simulink model "Matrix1_PP"  (Simulink 9.0)
settings: Solver=FixedStepDiscrete  StartTime=0.0  StopTime=19800  FixedStep=200  RelTol=1e-3  EnableMultiTasking=on
model workspace (MAT data in the model file):
  already_pp = 1
  input_dataset = Simulink.SimulationData.Dataset
  input_dataset.any.Name = ''
  input_dataset.any.Version = 3
  input_dataset.any.Storage = Simulink.SimulationData.Storage.RamDatasetStorage
  input_dataset.any.Storage.any.Version = 2
  input_dataset.any.Storage.any.Elements{1} = Simulink.SimulationData.Signal
  input_dataset.any.Storage.any.Elements{1}.Version = 1
  input_dataset.any.Storage.any.Elements{1}.Values = timeseries
  input_dataset.any.Storage.any.Elements{1}.Values.Name = 'unnamed'
  input_dataset.any.Storage.any.Elements{1}.Values.DataInfo = tsdata.datametadata
  input_dataset.any.Storage.any.Elements{1}.Values.DataInfo.Interpolation = tsdata.interpolation
  input_dataset.any.Storage.any.Elements{1}.Values.DataInfo.Interpolation.Fhandle : function handle (value not decoded)
  input_dataset.any.Storage.any.Elements{1}.Values.DataInfo.Interpolation.Name = 'linear'
  input_dataset.any.Storage.any.Elements{1}.Values.TimeInfo = tsdata.timemetadata
  input_dataset.any.Storage.any.Elements{1}.Values.TimeInfo.Length = 100
  input_dataset.any.Storage.any.Elements{1}.Values.TimeInfo.DuplicateTimes = 0
  input_dataset.any.Storage.any.Elements{1}.Values.TimeInfo.Time_ = [0; 200; 400; 600; 800; 1000; 1200; 1400; 1600; 1800; 2000; 2200; 2400; 2600; 2800; 3000; 3200; 3400; 3600; 3800; 4000; 4200; 4400; 4600; 4800; 5000; 5200; 5400; 5600; 5800; 6000; 6200; 6400; 6600; 6800; 7000; 7200; 7400; 7600; 7800; 8000; 8200; 8400; 8600; 8800; 9000; 9200; 9400; 9600; 9800; 10000; 10200; 10400; 10600; 10800; 11000; 11200; 11400; 11600; 11800; 12000; 12200; 12400; 12600; 12800; 13000; 13200; 13400; 13600; 13800; 14000; 14200; 14400; 14600; 14800; 15000; 15200; 15400; 15600; 15800; 16000; 16200; 16400; 16600; 16800; 17000; 17200; 17400; 17600; 17800; 18000; 18200; 18400; 18600; 18800; 19000; 19200; 19400; 19600; 19800]
  input_dataset.any.Storage.any.Elements{1}.Values.TimeInfo.Initialized = 1
  input_dataset.any.Storage.any.Elements{1}.Values.QualityInfo = tsdata.qualmetadata
  input_dataset.any.Storage.any.Elements{1}.Values.Data_ = [-264.228679452; 109.183142489; -274.5413175; -257.13272124; 12.9899054786; -241.961984531; 190.889132316; 190.528255248; 133.46375542; -210.080734513; 95.763151745; 11.1569655063; 283.784732858; 89.3948956274; 180.198345211; -27.7213747638; -40.5650977299; 195.188277241; -249.918111085; -220.097395436; -195.966832129; -65.4373186058; 198.827845703; 182.018634961; -263.717292498; -60.4453376319; 16.125498305; -49.9203192415; 94.1159345842; 76.7840155141; -124.809552023; -41.0092978508; -290.707724618; 290.438234627; -199.698954051; -236.270193043; -76.5541559667; -181.128958474; -6.18741719039; -96.3039519655; 270.978278867; 252.199223902; -268.393801392; 142.71485731; -138.528344161; -46.2986309947; 28.7225407289; 265.642190566; -49.35353741; 289.831479882; -119.127030773; 120.659253541; 99.8033109507; 23.4758790257; 118.863312108; 99.9167480416; -193.12052736; -223.191360168; 299.448236857; -197.327360186; -280.439507682; 36.7198756258; 229.119900271; 101.505182721; -185.740039692; -78.6500723617; -23.5644376438; 288.982770582; -206.157028664; 213.313683508; 86.8587221221; -74.2366738327; -185.445782858; -43.0482042124; -10.7867633809; -227.633032022; 53.704490817; -164.287392148; -69.2285253784; 49.7918296486; -148.916326517; -125.735601434; 70.2545306359; -140.831454114; 194.625760013; 289.598039833; 138.149275361; -93.673797531; 50.4415999671; -235.338590854; 243.78489039; 227.792234689; 190.656335622; -143.563200567; 56.6137503986; -286.492444356; -44.8444078715; -112.368667908; -203.109153413; -192.740287949]
  input_dataset.any.Storage.any.Elements{1}.Name = 'E'
settings Model: SuppressorTable=22 serialization::archive 11 0 6 0 0 0 0 0  Creator=scaife  LastModifiedBy=hbourbou  ExtModeAutoUpdateStatusClock=off
settings DataIOCC: ExternalInput=input_dataset  LimitDataPoints=on  LoadExternalInput=on  SaveFormat=Dataset  SignalLoggingSaveFormat=ModelDataLogs  SaveState=on  SignalLoggingName=sigsOut
settings DebuggingCC: AlgebraicLoopMsg=error  SaveWithParameterizedLinksMsg=none  SignalResolutionControl=TryResolveAllWithWarning  MultiTaskDSMMsg=warning  MultiTaskCondExecSysMsg=none  StrictBusMsg=None
settings HardwareCC: TargetUnknown=on
settings SFSimCC: SimParseCustomCode=off
settings GRTTargetCC: GeneratePreprocessorConditionals=Disable all  CombineOutputUpdateFcns=off  GRTInterface=on  ExtMode=on

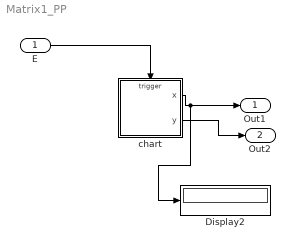
== system Matrix1_PP ==
  E : Inport
  Display2 : Display
  chart : Stateflow chart  TreatAsAtomicUnit=on
  Out1 : Outport
  Out2 : Outport  Port=2
  wires:
  E/1 -> chart/Trigger
  chart/1(x) -> Out1/1, Display2/1
  chart/2(y) -> Out2/1

== stateflow chart chart ==
  state A/
    en:
    i = 3;
    x(1) = x(2,i) + 1;
  state B/
    en:x(2) = x(2,2) + 1;
    y(2) = x(2) * 3;
  state C/
    en:x= y * 2;
  (default) -> A
  A -> B : E
  C -> A : E
  B -> C : E
  data: x output double size=[2 3] [0..100] =[1 2 3; 4 5 6]; i local int32; y output double size=[2 3] [0..100] =[1 2 3; 4 5 6]
  events: E input RISING_EDGE_EVENT
